simulink model "Sleep_Borbely"  (Simulink 6.4)
settings: Solver=ode45  StartTime=0.0  StopTime=3600*48  RelTol=1e-3
values from neighbouring files (symbols this model uses):
  Circadian_High = 0.90    (= 0.9)    [Respiratory_IC.m]    (also in State_UA_Khoo_IC.m)
  Circadian_Low = 0.15    [Respiratory_IC.m]    (also in State_UA_Khoo_IC.m)
  Circadian_Period = 24    [Respiratory_IC.m]    (also in State_UA_Khoo_IC.m)
  Circadian_Phase = 1.03*pi    (= 3.2358404332)    [Respiratory_IC.m]    (also in State_UA_Khoo_IC.m)
  fc = 0.4/60    (= 0.00666666666667)    [Respiratory_IC.m]    (also in State_UA_Khoo_IC.m)
  gc = 0.008/60    (= 0.000133333333333)    [Respiratory_IC.m]    (also in State_UA_Khoo_IC.m)
  Init_Proc_S = 0.90    (= 0.9)    [Respiratory_IC.m]    (also in State_UA_Khoo_IC.m)
  rc = 0.2/60    (= 0.00333333333333)    [Respiratory_IC.m]    (also in State_UA_Khoo_IC.m)
  Sleep = 0    [Respiratory_IC.m]    (also in State_UA_Khoo_IC.m)
  SWAo = 0.007    [Respiratory_IC.m]    (also in State_UA_Khoo_IC.m)
settings Model: LastModifiedBy=CLM
settings OptimizationCC: BlockReduction=off  BooleanDataType=off
settings DebuggingCC: SolverPrmCheckMsg=none  StrictBusMsg=None
settings HardwareCC: TargetUnknown=on

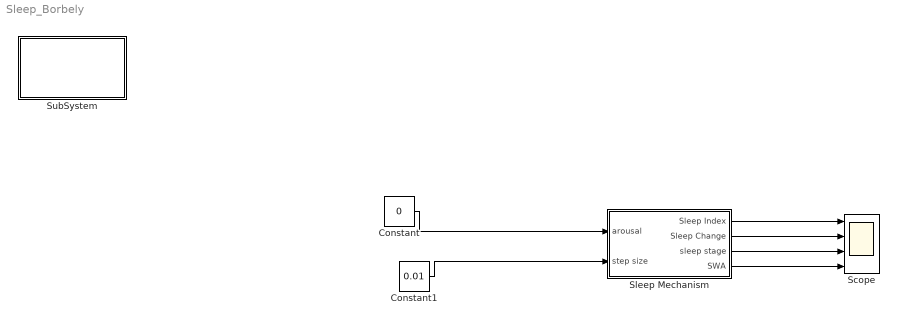
== system Sleep_Borbely ==
  Constant : Constant  Value=0  OutDataType=sfix(16)  ConRadixGroup=Use specified scaling  OutScaling=2^0  SampleTime=inf  FramePeriod=inf
  Constant1 : Constant  Value=0.01  OutDataType=sfix(16)  ConRadixGroup=Use specified scaling  OutScaling=2^0  SampleTime=inf  FramePeriod=inf
  Scope : Scope  NumInputPorts=4
      settings: YMin=-0.05~-0.05~-0.05~-0.05  YMax=1.05~1.05~1.05~1
  Sleep Mechanism : Subsystem
  SubSystem : Subsystem
      settings: OpenFcn=State_UA_Khoo_IC
      mask Display: disp('"double click here"\n to load \nState_UA_Khoo \ninitial values');
  wires:
  Constant1/1 -> Sleep Mechanism/2(step size)
  Constant/1 -> Sleep Mechanism/1(arousal)
  Sleep Mechanism/1(Sleep Index) -> Scope/1
  Sleep Mechanism/2(Sleep Change) -> Scope/2
  Sleep Mechanism/3(sleep stage) -> Scope/3
  Sleep Mechanism/4(SWA) -> Scope/4

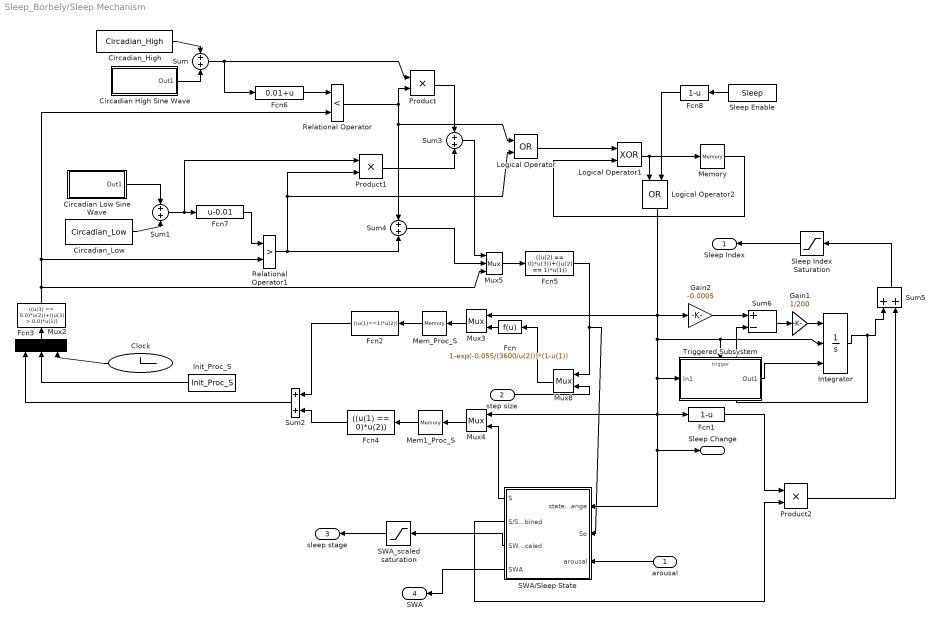
== system Sleep_Borbely/Sleep Mechanism ==
  arousal : Inport  Orientation=left
  step size : Inport  Port=2
  Circadian High Sine Wave : Subsystem
  Circadian Low Sine Wave : Subsystem
  Circadian_High : Constant  Value=Circadian_High  OutDataType=sfix(16)  ConRadixGroup=Use specified scaling  OutScaling=2^0  SampleTime=inf  FramePeriod=inf
  Circadian_Low : Constant  Value=Circadian_Low  OutDataType=sfix(16)  ConRadixGroup=Use specified scaling  OutScaling=2^0  SampleTime=inf  FramePeriod=inf
  Clock : Clock
      settings: Decimation=10
  Fcn : Fcn  Orientation=left  Expr=1-exp(-0.055/(3600/u(2)))*(1-u(1))
  Fcn1 : Fcn  Expr=1-u
  Fcn2 : Fcn  Orientation=left  Expr=((u(1)==1)*u(2))
  Fcn3 : Fcn  Orientation=up  Expr=((u(3) == 0.0)*u(2))+((u(3) > 0.0)*u(1))
  Fcn4 : Fcn  Orientation=left  Expr=((u(1) == 0)*u(2))
  Fcn5 : Fcn  Expr=((u(2) == 0)*u(3))+((u(2) == 1)*u(1))
  Fcn6 : Fcn  Expr=0.01+u
  Fcn7 : Fcn  Expr=u-0.01
  Fcn8 : Fcn  Orientation=left  Expr=1-u
  Gain1 : Gain  Gain=1/200  SaturateOnIntegerOverflow=on
  Gain2 : Gain  Gain=-0.0005  SaturateOnIntegerOverflow=on
  Init_Proc_S : Constant  Orientation=left  Value=Init_Proc_S  OutDataType=sfix(16)  ConRadixGroup=Use specified scaling  OutScaling=2^0  SampleTime=inf  FramePeriod=inf
  Integrator : Integrator  ExternalReset=rising  InitialConditionSource=external  InitialCondition=1
  Logical Operator : Logic  Operator=OR
  Logical Operator1 : Logic  Operator=XOR
  Logical Operator2 : Logic  Orientation=down  Operator=OR
  Mem1_Proc_S : Memory  Orientation=left  X0=0.9  InheritSampleTime=on
  Mem_Proc_S : Memory  Orientation=left  X0=0.9  InheritSampleTime=on
  Memory : Memory  X0=1  InheritSampleTime=on
  Mux2 : Mux  Orientation=up  Inputs=3
  Mux3 : Mux  Orientation=left  Inputs=2
  Mux4 : Mux  Orientation=left  Inputs=2
  Mux5 : Mux  Inputs=3
  Mux8 : Mux  Orientation=left  Inputs=2
  Product : Product  SaturateOnIntegerOverflow=on  RndMeth=Zero  InputSameDT=on
  Product1 : Product  SaturateOnIntegerOverflow=on  RndMeth=Zero  InputSameDT=on
  Product2 : Product  SaturateOnIntegerOverflow=on  RndMeth=Zero  InputSameDT=on
  Relational Operator : RelationalOperator  Operator=<  InputSameDT=on
  Relational Operator1 : RelationalOperator  Operator=>  InputSameDT=on
  SWA/Sleep State : Subsystem  Orientation=left
  SWA_scaled saturation : Saturate  Orientation=left  UpperLimit=1  LowerLimit=0
  Sleep Enable : Constant  Orientation=left  Value=Sleep  OutDataType=sfix(16)  ConRadixGroup=Use specified scaling  OutScaling=2^0  SampleTime=inf  FramePeriod=inf
  Sleep Index Saturation : Saturate  Orientation=left  UpperLimit=1  LowerLimit=0
  Sum{,1,3..4} (4 alike) : Sum  SaturateOnIntegerOverflow=on  InputSameDT=on
  Sum2 : Sum  Orientation=left  SaturateOnIntegerOverflow=on  InputSameDT=on
  Sum5 : Sum  Orientation=up  SaturateOnIntegerOverflow=on  InputSameDT=on
  Sum6 : Sum  Inputs=+-  SaturateOnIntegerOverflow=on  InputSameDT=on
  Triggered Subsystem : Subsystem  TreatAsAtomicUnit=on
  Sleep Index : Outport  Orientation=left
  Sleep Change : Outport  Port=2
  sleep stage : Outport  Orientation=left  Port=3
  SWA : Outport  Orientation=left  Port=4
  wires:
  arousal/1 -> SWA/Sleep State/3(arousal)
  Circadian_High/1 -> Sum/1
  Circadian Low Sine Wave/1(Out1) -> Sum1/1
  Circadian_Low/1 -> Sum1/2
  Sum/1 -> Fcn6/1, Product/1
  Sum1/1 -> Fcn7/1, Product1/1
  Logical Operator/1 -> Logical Operator1/1
  Memory/1 -> Logical Operator1/2
  Logical Operator1/1 -> Memory/1, Logical Operator2/1
  Relational Operator/1 -> Sum4/1, Logical Operator/1, Product/2
  Relational Operator1/1 -> Sum4/2, Logical Operator/2, Product1/2
  Product/1 -> Sum3/1
  Product1/1 -> Sum3/2
  Sum3/1 -> Mux5/1
  Mux2/1 -> Fcn3/1
  Init_Proc_S/1 -> Mux2/2
  Clock/1 -> Mux2/3
  Fcn2/1 -> Sum2/1
  Fcn4/1 -> Sum2/2
  Sum2/1 -> Mux2/1
  Fcn/1 -> Mux3/2
  SWA/Sleep State/1(S) -> Mux4/2
  Sum4/1 -> Mux5/2
  Mux5/1 -> Fcn5/1
  Mux3/1 -> Mem_Proc_S/1
  Mem_Proc_S/1 -> Fcn2/1
  Mux4/1 -> Mem1_Proc_S/1
  Fcn5/1 -> SWA/Sleep State/2(So), Mux8/1
  Mem1_Proc_S/1 -> Fcn4/1
  Fcn3/1 -> Relational Operator/2, Relational Operator1/2, Mux5/3
  Fcn6/1 -> Relational Operator/1
  Fcn7/1 -> Relational Operator1/1
  Mux8/1 -> Fcn/1
  step size/1 -> Mux8/2
  SWA/Sleep State/2(S/SWA Combined) -> Product2/2
  Fcn1/1 -> Product2/1
  Sum5/1 -> Sleep Index Saturation/1
  Product2/1 -> Sum5/2
  Sleep Index Saturation/1 -> Sleep Index/1
  Sleep Enable/1 -> Fcn8/1
  Fcn8/1 -> Logical Operator2/2
  Logical Operator2/1 -> Gain2/1, Mux3/1, Integrator/2, Triggered Subsystem/Trigger, Fcn1/1, Mux4/1, Sleep Change/1, SWA/Sleep State/1(state_change), Triggered Subsystem/1(In1)
  Integrator/1 -> Sum5/1, Sum6/2
  Triggered Subsystem/1(Out1) -> Integrator/3
  Gain2/1 -> Sum6/1
  Sum6/1 -> Gain1/1
  Gain1/1 -> Integrator/1
  Circadian High Sine Wave/1(Out1) -> Sum/2
  SWA/Sleep State/4(SWA) -> SWA/1
  SWA/Sleep State/3(SWA_scaled) -> SWA_scaled saturation/1
  SWA_scaled saturation/1 -> sleep stage/1

== system Sleep_Borbely/SubSystem ==

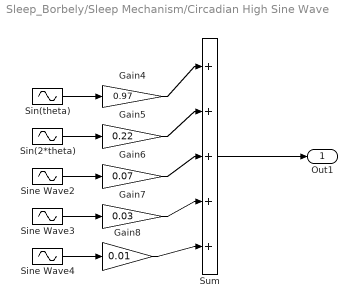
== system Sleep_Borbely/Sleep Mechanism/Circadian High Sine Wave ==
  Gain4 : Gain  Gain=0.97  SaturateOnIntegerOverflow=on
  Gain5 : Gain  Gain=0.22  SaturateOnIntegerOverflow=on
  Gain6 : Gain  Gain=0.07  SaturateOnIntegerOverflow=on
  Gain7 : Gain  Gain=0.03  SaturateOnIntegerOverflow=on
  Gain8 : Gain  Gain=0.01  SaturateOnIntegerOverflow=on
  Sin(2*theta) : Sin  Amplitude=0.12  Frequency=(2*2*pi)/(Circadian_Period*3600)  Phase=Circadian_Phase  SampleTime=0
  Sin(theta) : Sin  Amplitude=0.12  Frequency=(2*pi)/(Circadian_Period*3600)  Phase=Circadian_Phase  SampleTime=0
  Sine Wave2 : Sin  Amplitude=0.12  Frequency=(3*2*pi)/(Circadian_Period*3600)  Phase=Circadian_Phase  SampleTime=0
  Sine Wave3 : Sin  Amplitude=0.12  Frequency=(4*2*pi)/(Circadian_Period*3600)  Phase=Circadian_Phase  SampleTime=0
  Sine Wave4 : Sin  Amplitude=0.12  Frequency=(5*2*pi)/(Circadian_Period*3600)  Phase=Circadian_Phase  SampleTime=0
  Sum : Sum  Inputs=|+++++  SaturateOnIntegerOverflow=on  InputSameDT=on
  Out1 : Outport
  wires:
  Sin(theta)/1 -> Gain4/1
  Gain4/1 -> Sum/1
  Sin(2*theta)/1 -> Gain5/1
  Gain5/1 -> Sum/2
  Sine Wave2/1 -> Gain6/1
  Gain6/1 -> Sum/3
  Sine Wave3/1 -> Gain7/1
  Gain7/1 -> Sum/4
  Sine Wave4/1 -> Gain8/1
  Gain8/1 -> Sum/5
  Sum/1 -> Out1/1

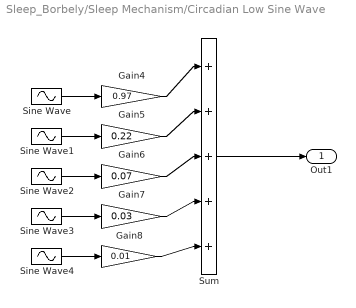
== system Sleep_Borbely/Sleep Mechanism/Circadian Low Sine Wave ==
  Gain4 : Gain  Gain=0.97  SaturateOnIntegerOverflow=on
  Gain5 : Gain  Gain=0.22  SaturateOnIntegerOverflow=on
  Gain6 : Gain  Gain=0.07  SaturateOnIntegerOverflow=on
  Gain7 : Gain  Gain=0.03  SaturateOnIntegerOverflow=on
  Gain8 : Gain  Gain=0.01  SaturateOnIntegerOverflow=on
  Sine Wave : Sin  Amplitude=0.12  Frequency=(2*pi)/(Circadian_Period*3600)  Phase=Circadian_Phase  SampleTime=0  VectorParams1D=off
  Sine Wave1 : Sin  Amplitude=0.12  Frequency=(2*2*pi)/(Circadian_Period*3600)  Phase=Circadian_Period  SampleTime=0
  Sine Wave2 : Sin  Amplitude=0.12  Frequency=(3*2*pi)/(Circadian_Period*3600)  Phase=Circadian_Phase  SampleTime=0
  Sine Wave3 : Sin  Amplitude=0.12  Frequency=(4*2*pi)/(Circadian_Period*3600)  Phase=Circadian_Phase  SampleTime=0
  Sine Wave4 : Sin  Amplitude=0.12  Frequency=(5*2*pi)/(Circadian_Period*3600)  Phase=Circadian_Phase  SampleTime=0
  Sum : Sum  Inputs=|+++++  SaturateOnIntegerOverflow=on  InputSameDT=on
  Out1 : Outport
  wires:
  Sum/1 -> Out1/1
  Gain8/1 -> Sum/5
  Sine Wave4/1 -> Gain8/1
  Gain7/1 -> Sum/4
  Sine Wave3/1 -> Gain7/1
  Gain6/1 -> Sum/3
  Sine Wave2/1 -> Gain6/1
  Gain5/1 -> Sum/2
  Sine Wave1/1 -> Gain5/1
  Gain4/1 -> Sum/1
  Sine Wave/1 -> Gain4/1

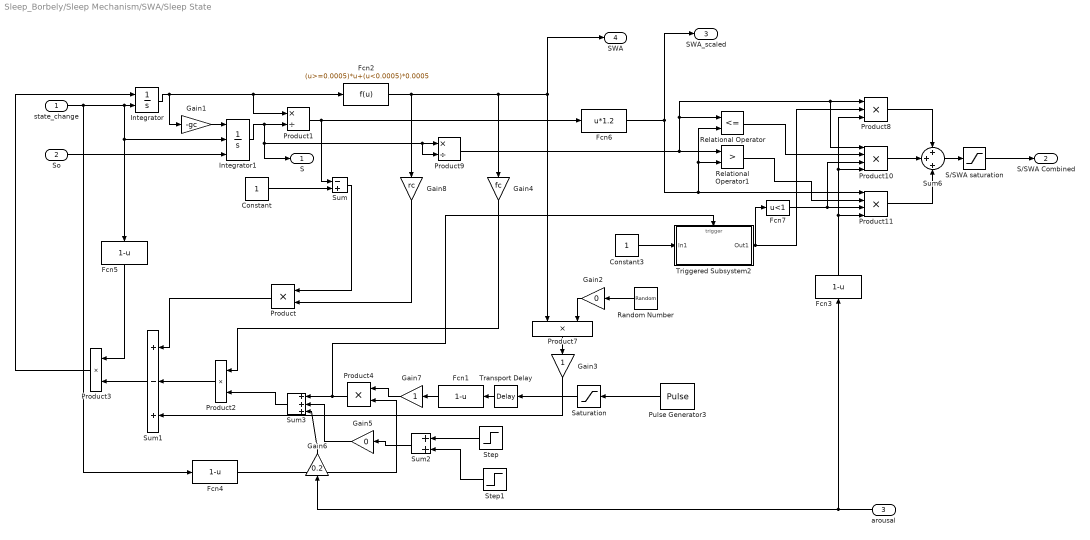
== system Sleep_Borbely/Sleep Mechanism/SWA/Sleep State ==
  state_change : Inport
  So : Inport  Port=2
  arousal : Inport  Orientation=left  Port=3
  Constant : Constant  Value=1  OutDataType=sfix(16)  ConRadixGroup=Use specified scaling  OutScaling=2^0  SampleTime=inf  FramePeriod=inf
  Constant3 : Constant  Value=1  OutDataType=sfix(16)  ConRadixGroup=Use specified scaling  OutScaling=2^0  SampleTime=inf  FramePeriod=inf
  Fcn1 : Fcn  Orientation=left  Expr=1-u
  Fcn2 : Fcn  Expr=(u>=0.0005)*u+(u<0.0005)*0.0005
  Fcn3 : Fcn  Orientation=up  Expr=1-u
  Fcn4 : Fcn  Expr=1-u
  Fcn5 : Fcn  Orientation=down  Expr=1-u
  Fcn6 : Fcn  Expr=u*1.2
  Fcn7 : Fcn  Expr=u<1
  Gain1 : Gain  Gain=-gc  SaturateOnIntegerOverflow=on
  Gain2 : Gain  Orientation=left  Gain=0  SaturateOnIntegerOverflow=on
  Gain3 : Gain  Orientation=down  SaturateOnIntegerOverflow=on
  Gain4 : Gain  Orientation=down  Gain=fc  SaturateOnIntegerOverflow=on
  Gain5 : Gain  Orientation=left  Gain=0  SaturateOnIntegerOverflow=on
  Gain6 : Gain  Orientation=up  Gain=0.2  SaturateOnIntegerOverflow=on
  Gain7 : Gain  Orientation=left  SaturateOnIntegerOverflow=on
  Gain8 : Gain  Orientation=down  Gain=rc  SaturateOnIntegerOverflow=on
  Integrator : Integrator  ExternalReset=either  InitialCondition=SWAo  LimitOutput=on
  Integrator1 : Integrator  ExternalReset=falling  InitialConditionSource=external  InitialCondition=0.8  LimitOutput=on
  Product : Product  Orientation=left  SaturateOnIntegerOverflow=on  RndMeth=Zero  InputSameDT=on
  Product1 : Product  Inputs=*/  SaturateOnIntegerOverflow=on  RndMeth=Zero  InputSameDT=on
  Product10 : Product  Inputs=4  SaturateOnIntegerOverflow=on  RndMeth=Zero  InputSameDT=on
  Product11 : Product  Inputs=4  SaturateOnIntegerOverflow=on  RndMeth=Zero  InputSameDT=on
  Product2 : Product  Orientation=left  SaturateOnIntegerOverflow=on  RndMeth=Zero  InputSameDT=on
  Product3 : Product  Orientation=left  SaturateOnIntegerOverflow=on  RndMeth=Zero  InputSameDT=on
  Product4 : Product  Orientation=left  Inputs=**  SaturateOnIntegerOverflow=on  RndMeth=Zero  InputSameDT=on
  Product7 : Product  Orientation=down  SaturateOnIntegerOverflow=on  RndMeth=Zero  InputSameDT=on
  Product8 : Product  Inputs=3  SaturateOnIntegerOverflow=on  RndMeth=Zero  InputSameDT=on
  Product9 : Product  Inputs=*/  SaturateOnIntegerOverflow=on  RndMeth=Zero  InputSameDT=on
  Pulse Generator3 : DiscretePulseGenerator  Orientation=left  PulseType=Time based  Period=3600*1.8  PulseWidth=85
  Random Number : RandomNumber  Orientation=left  Variance=0.01  Seed=0.005  SampleTime=0
  Relational Operator : RelationalOperator  Operator=<=  InputSameDT=on
  Relational Operator1 : RelationalOperator  Operator=>  InputSameDT=on
  S/SWA saturation : Saturate  UpperLimit=1  LowerLimit=0
  Saturation : Saturate  Orientation=left  UpperLimit=1  LowerLimit=0
  Step : Step  Orientation=left  Time=3600  SampleTime=0
  Step1 : Step  Orientation=left  Time=3600+4  After=-1  SampleTime=0
  Sum : Sum  Inputs=-+  SaturateOnIntegerOverflow=on  InputSameDT=on
  Sum1 : Sum  Orientation=left  Inputs=+-+  SaturateOnIntegerOverflow=on  InputSameDT=on
  Sum2 : Sum  Orientation=left  SaturateOnIntegerOverflow=on  InputSameDT=on
  Sum3 : Sum  Orientation=left  Inputs=+++  SaturateOnIntegerOverflow=on  InputSameDT=on
  Sum6 : Sum  Inputs=+++  SaturateOnIntegerOverflow=on  InputSameDT=on
  Transport Delay : TransportDelay  Orientation=left  DelayTime=5  InitialOutput=1  BufferSize=1024*10
  Triggered Subsystem2 : Subsystem  TreatAsAtomicUnit=on
  S : Outport
  S/SWA Combined : Outport  Port=2
  SWA_scaled : Outport  Port=3
  SWA : Outport  Port=4
  wires:
  Relational Operator1/1 -> Product11/2
  Fcn7/1 -> Product11/3, Product10/3
  Product10/1 -> Sum6/2
  Product11/1 -> Sum6/3
  Relational Operator/1 -> Product10/2
  Sum6/1 -> S/SWA saturation/1
  Product8/1 -> Sum6/1
  Triggered Subsystem2/1(Out1) -> Product8/2, Fcn7/1
  Constant3/1 -> Triggered Subsystem2/1(In1)
  Gain2/1 -> Product7/2
  Saturation/1 -> Transport Delay/1
  Random Number/1 -> Gain2/1
  Product7/1 -> Gain3/1
  Gain6/1 -> Sum3/3
  Gain5/1 -> Sum3/2
  arousal/1 -> Gain6/1, Fcn3/1
  Sum3/1 -> Product2/2
  Sum2/1 -> Gain5/1
  Step1/1 -> Sum2/2
  Step/1 -> Sum2/1
  Transport Delay/1 -> Fcn1/1
  Constant/1 -> Sum/2
  Product1/1 -> Sum/1, Fcn6/1
  Gain1/1 -> Integrator1/1
  Integrator/1 -> Product1/1, Fcn2/1, Gain1/1
  Sum/1 -> Product/1
  Product/1 -> Sum1/1
  Product2/1 -> Sum1/2
  Gain3/1 -> Sum1/3
  Integrator1/1 -> Product1/2, S/1, Product9/1, Product9/2
  state_change/1 -> Integrator1/2, Fcn5/1, Integrator/2, Fcn4/1
  So/1 -> Integrator1/3
  Fcn2/1 -> Gain4/1, Product7/1, SWA/1, Gain8/1
  Fcn6/1 -> Relational Operator1/2, Relational Operator/2, Product11/1, SWA_scaled/1
  Product9/1 -> Relational Operator1/1, Relational Operator/1, Product8/1, Product10/1
  S/SWA saturation/1 -> S/SWA Combined/1
  Gain4/1 -> Product2/1
  Gain8/1 -> Product/2
  Fcn1/1 -> Gain7/1
  Sum1/1 -> Product3/2
  Product3/1 -> Integrator/1
  Fcn5/1 -> Product3/1
  Pulse Generator3/1 -> Saturation/1
  Fcn3/1 -> Product8/3, Product10/4, Product11/4
  Gain7/1 -> Product4/1
  Fcn4/1 -> Product4/2
  Product4/1 -> Sum3/1, Triggered Subsystem2/Trigger

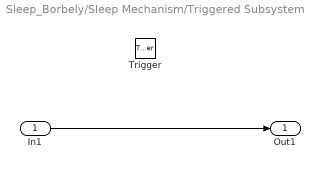
== system Sleep_Borbely/Sleep Mechanism/Triggered Subsystem ==
  In1 : Inport
  Trigger : TriggerPort
  Out1 : Outport
  wires:
  In1/1 -> Out1/1

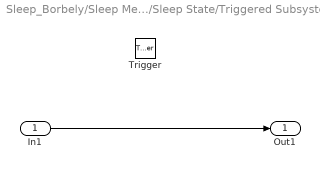
== system Sleep_Borbely/Sleep Mechanism/SWA/Sleep State/Triggered Subsystem2 ==
  In1 : Inport
  Trigger : TriggerPort
  Out1 : Outport
  wires:
  In1/1 -> Out1/1
